simulink model "System"  (R2020a)
settings: Solver=VariableStepAuto  StartTime=0.0  StopTime=30000  RelTol=1e-3
values from neighbouring files (symbols this model uses):
  params = struct()    [LOAD_PARAMS.m]
libraries: simulink x25
(part 2 of 2)

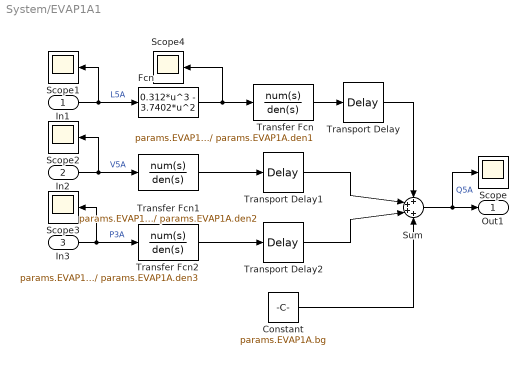
== system System/EVAP1A1 ==
  In1 : Inport
  In2 : Inport  Port=2
  In3 : Inport  Port=3
  Constant : Constant  Value=params.EVAP1A.bg
  Fcn : Fcn  Expr=0.312*u^3 - 3.7402*u^2
  Scope{,1..4} (5 alike) : Scope
  Sum : Sum  Inputs=++++
  Transfer Fcn : TransferFcn  Numerator=params.EVAP1A.num1  Denominator=params.EVAP1A.den1
  Transfer Fcn1 : TransferFcn  Numerator=params.EVAP1A.num2  Denominator=params.EVAP1A.den2
  Transfer Fcn2 : TransferFcn  Numerator=params.EVAP1A.num3  Denominator=params.EVAP1A.den3
  Transport Delay : TransportDelay  DelayTime=params.EVAP1A.td1
  Transport Delay1 : TransportDelay  DelayTime=params.EVAP1A.td2
  Transport Delay2 : TransportDelay  DelayTime=params.EVAP1A.td3
  Out1 : Outport
  wires:
  Transfer Fcn/1 -> Transport Delay/1
  Transfer Fcn1/1 -> Transport Delay1/1
  Transfer Fcn2/1 -> Transport Delay2/1
  In1/1 -> Fcn/1, Scope1/1  "L5A"
  In2/1 -> Scope2/1, Transfer Fcn1/1  "V5A"
  In3/1 -> Scope3/1, Transfer Fcn2/1  "P3A"
  Sum/1 -> Scope/1, Out1/1  "Q5A"
  Constant/1 -> Sum/4
  Fcn/1 -> Scope4/1, Transfer Fcn/1
  Transport Delay/1 -> Sum/1
  Transport Delay1/1 -> Sum/2
  Transport Delay2/1 -> Sum/3

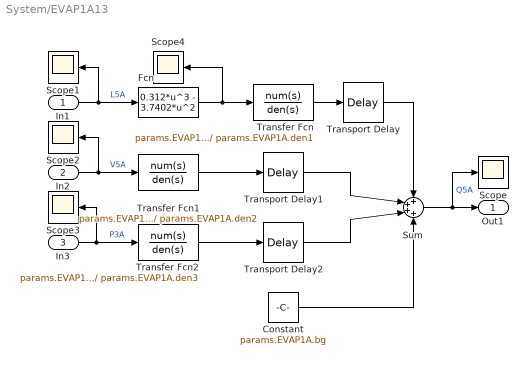
== system System/EVAP1A13 ==
  In1 : Inport
  In2 : Inport  Port=2
  In3 : Inport  Port=3
  Constant : Constant  Value=params.EVAP1A.bg
  Fcn : Fcn  Expr=0.312*u^3 - 3.7402*u^2
  Scope{,1..4} (5 alike) : Scope
  Sum : Sum  Inputs=++++
  Transfer Fcn : TransferFcn  Numerator=params.EVAP1A.num1  Denominator=params.EVAP1A.den1
  Transfer Fcn1 : TransferFcn  Numerator=params.EVAP1A.num2  Denominator=params.EVAP1A.den2
  Transfer Fcn2 : TransferFcn  Numerator=params.EVAP1A.num3  Denominator=params.EVAP1A.den3
  Transport Delay : TransportDelay  DelayTime=params.EVAP1A.td1
  Transport Delay1 : TransportDelay  DelayTime=params.EVAP1A.td2
  Transport Delay2 : TransportDelay  DelayTime=params.EVAP1A.td3
  Out1 : Outport
  wires:
  Transfer Fcn/1 -> Transport Delay/1
  Transfer Fcn1/1 -> Transport Delay1/1
  Transfer Fcn2/1 -> Transport Delay2/1
  In1/1 -> Fcn/1, Scope1/1  "L5A"
  In2/1 -> Scope2/1, Transfer Fcn1/1  "V5A"
  In3/1 -> Scope3/1, Transfer Fcn2/1  "P3A"
  Sum/1 -> Scope/1, Out1/1  "Q5A"
  Constant/1 -> Sum/4
  Fcn/1 -> Scope4/1, Transfer Fcn/1
  Transport Delay/1 -> Sum/1
  Transport Delay1/1 -> Sum/2
  Transport Delay2/1 -> Sum/3

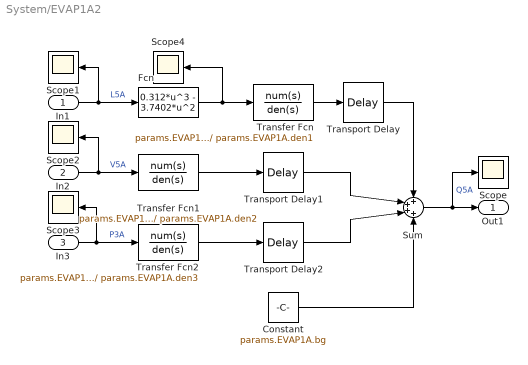
== system System/EVAP1A2 ==
  In1 : Inport
  In2 : Inport  Port=2
  In3 : Inport  Port=3
  Constant : Constant  Value=params.EVAP1A.bg
  Fcn : Fcn  Expr=0.312*u^3 - 3.7402*u^2
  Scope{,1..4} (5 alike) : Scope
  Sum : Sum  Inputs=++++
  Transfer Fcn : TransferFcn  Numerator=params.EVAP1A.num1  Denominator=params.EVAP1A.den1
  Transfer Fcn1 : TransferFcn  Numerator=params.EVAP1A.num2  Denominator=params.EVAP1A.den2
  Transfer Fcn2 : TransferFcn  Numerator=params.EVAP1A.num3  Denominator=params.EVAP1A.den3
  Transport Delay : TransportDelay  DelayTime=params.EVAP1A.td1
  Transport Delay1 : TransportDelay  DelayTime=params.EVAP1A.td2
  Transport Delay2 : TransportDelay  DelayTime=params.EVAP1A.td3
  Out1 : Outport
  wires:
  Transfer Fcn/1 -> Transport Delay/1
  Transfer Fcn1/1 -> Transport Delay1/1
  Transfer Fcn2/1 -> Transport Delay2/1
  In1/1 -> Fcn/1, Scope1/1  "L5A"
  In2/1 -> Scope2/1, Transfer Fcn1/1  "V5A"
  In3/1 -> Scope3/1, Transfer Fcn2/1  "P3A"
  Sum/1 -> Scope/1, Out1/1  "Q5A"
  Constant/1 -> Sum/4
  Fcn/1 -> Scope4/1, Transfer Fcn/1
  Transport Delay/1 -> Sum/1
  Transport Delay1/1 -> Sum/2
  Transport Delay2/1 -> Sum/3

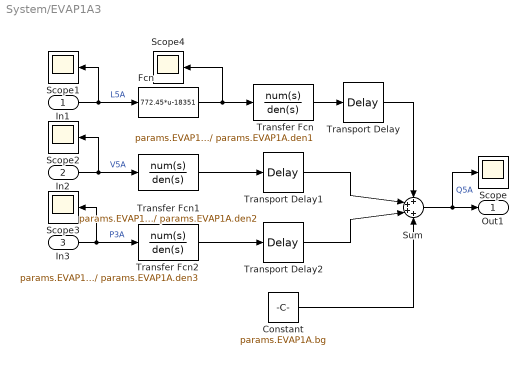
== system System/EVAP1A3 ==
  In1 : Inport
  In2 : Inport  Port=2
  In3 : Inport  Port=3
  Constant : Constant  Value=params.EVAP1A.bg
  Fcn : Fcn  Expr=772.45*u-18351
  Scope{,1..4} (5 alike) : Scope
  Sum : Sum  Inputs=++++
  Transfer Fcn : TransferFcn  Numerator=params.EVAP1A.num1  Denominator=params.EVAP1A.den1
  Transfer Fcn1 : TransferFcn  Numerator=params.EVAP1A.num2  Denominator=params.EVAP1A.den2
  Transfer Fcn2 : TransferFcn  Numerator=params.EVAP1A.num3  Denominator=params.EVAP1A.den3
  Transport Delay : TransportDelay  DelayTime=params.EVAP1A.td1
  Transport Delay1 : TransportDelay  DelayTime=params.EVAP1A.td2
  Transport Delay2 : TransportDelay  DelayTime=params.EVAP1A.td3
  Out1 : Outport
  wires:
  Transfer Fcn/1 -> Transport Delay/1
  Transfer Fcn1/1 -> Transport Delay1/1
  Transfer Fcn2/1 -> Transport Delay2/1
  In1/1 -> Fcn/1, Scope1/1  "L5A"
  In2/1 -> Scope2/1, Transfer Fcn1/1  "V5A"
  In3/1 -> Scope3/1, Transfer Fcn2/1  "P3A"
  Sum/1 -> Scope/1, Out1/1  "Q5A"
  Constant/1 -> Sum/4
  Fcn/1 -> Scope4/1, Transfer Fcn/1
  Transport Delay/1 -> Sum/1
  Transport Delay1/1 -> Sum/2
  Transport Delay2/1 -> Sum/3

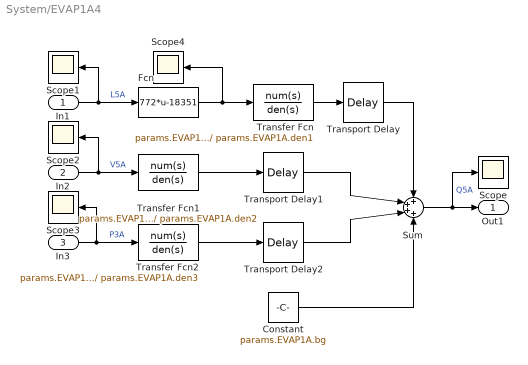
== system System/EVAP1A4 ==
  In1 : Inport
  In2 : Inport  Port=2
  In3 : Inport  Port=3
  Constant : Constant  Value=params.EVAP1A.bg
  Fcn : Fcn  Expr=772*u-18351
  Scope{,1..4} (5 alike) : Scope
  Sum : Sum  Inputs=++++
  Transfer Fcn : TransferFcn  Numerator=params.EVAP1A.num1  Denominator=params.EVAP1A.den1
  Transfer Fcn1 : TransferFcn  Numerator=params.EVAP1A.num2  Denominator=params.EVAP1A.den2
  Transfer Fcn2 : TransferFcn  Numerator=params.EVAP1A.num3  Denominator=params.EVAP1A.den3
  Transport Delay : TransportDelay  DelayTime=params.EVAP1A.td1
  Transport Delay1 : TransportDelay  DelayTime=params.EVAP1A.td2
  Transport Delay2 : TransportDelay  DelayTime=params.EVAP1A.td3
  Out1 : Outport
  wires:
  Transfer Fcn/1 -> Transport Delay/1
  Transfer Fcn1/1 -> Transport Delay1/1
  Transfer Fcn2/1 -> Transport Delay2/1
  In1/1 -> Fcn/1, Scope1/1  "L5A"
  In2/1 -> Scope2/1, Transfer Fcn1/1  "V5A"
  In3/1 -> Scope3/1, Transfer Fcn2/1  "P3A"
  Sum/1 -> Scope/1, Out1/1  "Q5A"
  Constant/1 -> Sum/4
  Fcn/1 -> Scope4/1, Transfer Fcn/1
  Transport Delay/1 -> Sum/1
  Transport Delay1/1 -> Sum/2
  Transport Delay2/1 -> Sum/3

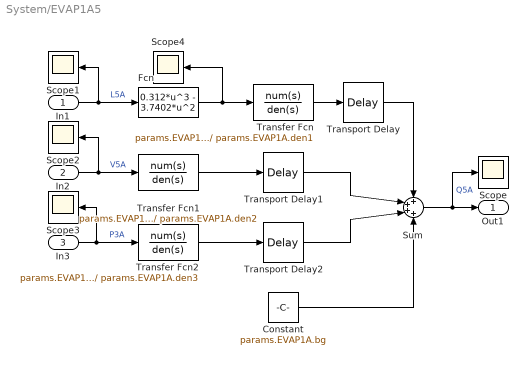
== system System/EVAP1A5 ==
  In1 : Inport
  In2 : Inport  Port=2
  In3 : Inport  Port=3
  Constant : Constant  Value=params.EVAP1A.bg
  Fcn : Fcn  Expr=0.312*u^3 - 3.7402*u^2
  Scope{,1..4} (5 alike) : Scope
  Sum : Sum  Inputs=++++
  Transfer Fcn : TransferFcn  Numerator=params.EVAP1A.num1  Denominator=params.EVAP1A.den1
  Transfer Fcn1 : TransferFcn  Numerator=params.EVAP1A.num2  Denominator=params.EVAP1A.den2
  Transfer Fcn2 : TransferFcn  Numerator=params.EVAP1A.num3  Denominator=params.EVAP1A.den3
  Transport Delay : TransportDelay  DelayTime=params.EVAP1A.td1
  Transport Delay1 : TransportDelay  DelayTime=params.EVAP1A.td2
  Transport Delay2 : TransportDelay  DelayTime=params.EVAP1A.td3
  Out1 : Outport
  wires:
  Transfer Fcn/1 -> Transport Delay/1
  Transfer Fcn1/1 -> Transport Delay1/1
  Transfer Fcn2/1 -> Transport Delay2/1
  In1/1 -> Fcn/1, Scope1/1  "L5A"
  In2/1 -> Scope2/1, Transfer Fcn1/1  "V5A"
  In3/1 -> Scope3/1, Transfer Fcn2/1  "P3A"
  Sum/1 -> Scope/1, Out1/1  "Q5A"
  Constant/1 -> Sum/4
  Fcn/1 -> Scope4/1, Transfer Fcn/1
  Transport Delay/1 -> Sum/1
  Transport Delay1/1 -> Sum/2
  Transport Delay2/1 -> Sum/3

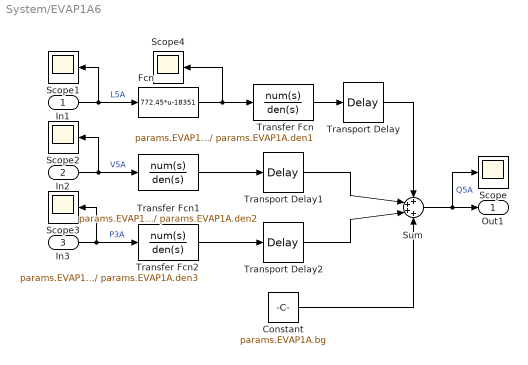
== system System/EVAP1A6 ==
  In1 : Inport
  In2 : Inport  Port=2
  In3 : Inport  Port=3
  Constant : Constant  Value=params.EVAP1A.bg
  Fcn : Fcn  Expr=772.45*u-18351
  Scope{,1..4} (5 alike) : Scope
  Sum : Sum  Inputs=++++
  Transfer Fcn : TransferFcn  Numerator=params.EVAP1A.num1  Denominator=params.EVAP1A.den1
  Transfer Fcn1 : TransferFcn  Numerator=params.EVAP1A.num2  Denominator=params.EVAP1A.den2
  Transfer Fcn2 : TransferFcn  Numerator=params.EVAP1A.num3  Denominator=params.EVAP1A.den3
  Transport Delay : TransportDelay  DelayTime=params.EVAP1A.td1
  Transport Delay1 : TransportDelay  DelayTime=params.EVAP1A.td2
  Transport Delay2 : TransportDelay  DelayTime=params.EVAP1A.td3
  Out1 : Outport
  wires:
  Transfer Fcn/1 -> Transport Delay/1
  Transfer Fcn1/1 -> Transport Delay1/1
  Transfer Fcn2/1 -> Transport Delay2/1
  In1/1 -> Fcn/1, Scope1/1  "L5A"
  In2/1 -> Scope2/1, Transfer Fcn1/1  "V5A"
  In3/1 -> Scope3/1, Transfer Fcn2/1  "P3A"
  Sum/1 -> Scope/1, Out1/1  "Q5A"
  Constant/1 -> Sum/4
  Fcn/1 -> Scope4/1, Transfer Fcn/1
  Transport Delay/1 -> Sum/1
  Transport Delay1/1 -> Sum/2
  Transport Delay2/1 -> Sum/3

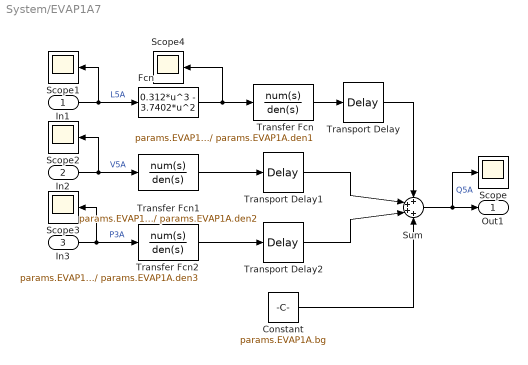
== system System/EVAP1A7 ==
  In1 : Inport
  In2 : Inport  Port=2
  In3 : Inport  Port=3
  Constant : Constant  Value=params.EVAP1A.bg
  Fcn : Fcn  Expr=0.312*u^3 - 3.7402*u^2
  Scope{,1..4} (5 alike) : Scope
  Sum : Sum  Inputs=++++
  Transfer Fcn : TransferFcn  Numerator=params.EVAP1A.num1  Denominator=params.EVAP1A.den1
  Transfer Fcn1 : TransferFcn  Numerator=params.EVAP1A.num2  Denominator=params.EVAP1A.den2
  Transfer Fcn2 : TransferFcn  Numerator=params.EVAP1A.num3  Denominator=params.EVAP1A.den3
  Transport Delay : TransportDelay  DelayTime=params.EVAP1A.td1
  Transport Delay1 : TransportDelay  DelayTime=params.EVAP1A.td2
  Transport Delay2 : TransportDelay  DelayTime=params.EVAP1A.td3
  Out1 : Outport
  wires:
  Transfer Fcn/1 -> Transport Delay/1
  Transfer Fcn1/1 -> Transport Delay1/1
  Transfer Fcn2/1 -> Transport Delay2/1
  In1/1 -> Fcn/1, Scope1/1  "L5A"
  In2/1 -> Scope2/1, Transfer Fcn1/1  "V5A"
  In3/1 -> Scope3/1, Transfer Fcn2/1  "P3A"
  Sum/1 -> Scope/1, Out1/1  "Q5A"
  Constant/1 -> Sum/4
  Fcn/1 -> Scope4/1, Transfer Fcn/1
  Transport Delay/1 -> Sum/1
  Transport Delay1/1 -> Sum/2
  Transport Delay2/1 -> Sum/3

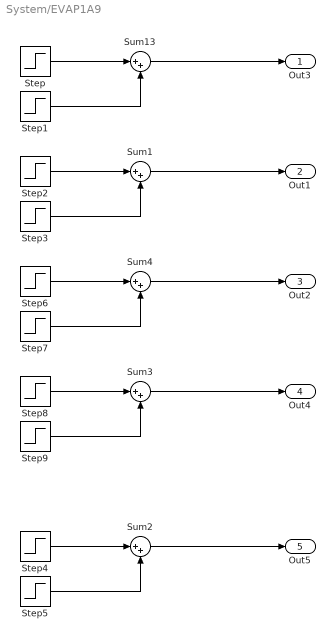
== system System/EVAP1A9 ==
  Step : Step  Time=1000  Before=200  After=0  SampleTime=0
  Step1 : Step  Time=2000  After=200  SampleTime=0
  Step2 : Step  Time=1000  Before=2  After=0  SampleTime=0
  Step3 : Step  Time=2000  After=2  SampleTime=0
  Step4 : Step  Time=1000  Before=74  After=72  SampleTime=0
  Step5 : Step  Time=2000  After=2  SampleTime=0
  Step6 : Step  Time=3000  Before=200  After=0  SampleTime=0
  Step7 : Step  Time=4000  After=200  SampleTime=0
  Step8 : Step  Time=3000  Before=2  After=0  SampleTime=0
  Step9 : Step  Time=4000  After=2  SampleTime=0
  Sum{1..4,13} (5 alike) : Sum  Inputs=|++
  Out3 : Outport
  Out1 : Outport  Port=2
  Out2 : Outport  Port=3
  Out4 : Outport  Port=4
  Out5 : Outport  Port=5
  wires:
  Step1/1 -> Sum13/2
  Step/1 -> Sum13/1
  Sum13/1 -> Out3/1
  Step2/1 -> Sum1/1
  Sum1/1 -> Out1/1
  Step3/1 -> Sum1/2
  Step4/1 -> Sum2/1
  Sum2/1 -> Out5/1
  Step5/1 -> Sum2/2
  Sum4/1 -> Out2/1
  Step6/1 -> Sum4/1
  Step9/1 -> Sum3/2
  Step8/1 -> Sum3/1
  Sum3/1 -> Out4/1
  Step7/1 -> Sum4/2

== system System/EVAP2A ==
  In1 : Inport
  In2 : Inport  Port=2
  In3 : Inport  Port=3
  Constant : Constant  Value=params.EVAP1A.bg
  Fcn : Fcn  Expr=0.312*u^3 - 3.7402*u^2
  Scope{,1..3} (4 alike) : Scope
  Sum : Sum  Inputs=++++
  Transfer Fcn : TransferFcn  Numerator=params.EVAP1A.num1  Denominator=params.EVAP1A.den1
  Transfer Fcn1 : TransferFcn  Numerator=params.EVAP1A.num2  Denominator=params.EVAP1A.den2
  Transfer Fcn2 : TransferFcn  Numerator=params.EVAP1A.num3  Denominator=params.EVAP1A.den3
  Transport Delay : TransportDelay  DelayTime=params.EVAP1A.td1
  Transport Delay1 : TransportDelay  DelayTime=params.EVAP1A.td3
  Transport Delay2 : TransportDelay  DelayTime=params.EVAP1A.td2
  Out1 : Outport
  wires:
  Transfer Fcn/1 -> Transport Delay/1
  Transfer Fcn1/1 -> Transport Delay2/1
  Transfer Fcn2/1 -> Transport Delay1/1
  In1/1 -> Fcn/1, Scope1/1  "L6A"
  In2/1 -> Scope2/1, Transfer Fcn1/1  "V6A"
  In3/1 -> Scope3/1, Transfer Fcn2/1  "P3A"
  Sum/1 -> Scope/1, Out1/1  "Q5A"
  Constant/1 -> Sum/4
  Fcn/1 -> Transfer Fcn/1
  Transport Delay/1 -> Sum/1
  Transport Delay2/1 -> Sum/2
  Transport Delay1/1 -> Sum/3

== system System/EVAP2A1 ==
  In1 : Inport
  In2 : Inport  Port=2
  In3 : Inport  Port=3
  Constant : Constant  Value=params.EVAP1A.bg
  Fcn : Fcn  Expr=0.312*u^3 - 3.7402*u^2
  Scope{,1..3} (4 alike) : Scope
  Sum : Sum  Inputs=++++
  Transfer Fcn : TransferFcn  Numerator=params.EVAP1A.num1  Denominator=params.EVAP1A.den1
  Transfer Fcn1 : TransferFcn  Numerator=params.EVAP1A.num2  Denominator=params.EVAP1A.den2
  Transfer Fcn2 : TransferFcn  Numerator=params.EVAP1A.num3  Denominator=params.EVAP1A.den3
  Transport Delay : TransportDelay  DelayTime=params.EVAP1A.td1
  Transport Delay1 : TransportDelay  DelayTime=params.EVAP1A.td3
  Transport Delay2 : TransportDelay  DelayTime=params.EVAP1A.td2
  Out1 : Outport
  wires:
  Transfer Fcn/1 -> Transport Delay/1
  Transfer Fcn1/1 -> Transport Delay2/1
  Transfer Fcn2/1 -> Transport Delay1/1
  In1/1 -> Fcn/1, Scope1/1  "L6A"
  In2/1 -> Scope2/1, Transfer Fcn1/1  "V6A"
  In3/1 -> Scope3/1, Transfer Fcn2/1  "P3A"
  Sum/1 -> Scope/1, Out1/1  "Q5A"
  Constant/1 -> Sum/4
  Fcn/1 -> Transfer Fcn/1
  Transport Delay/1 -> Sum/1
  Transport Delay2/1 -> Sum/2
  Transport Delay1/1 -> Sum/3

== system System/EVAP2A3 ==
  In1 : Inport
  In2 : Inport  Port=2
  In3 : Inport  Port=3
  Constant : Constant  Value=params.EVAP1A.bg
  Fcn : Fcn  Expr=772.45*u-18351
  Scope{,1..3} (4 alike) : Scope
  Sum : Sum  Inputs=++++
  Transfer Fcn : TransferFcn  Numerator=params.EVAP1A.num1  Denominator=params.EVAP1A.den1
  Transfer Fcn1 : TransferFcn  Numerator=params.EVAP1A.num2  Denominator=params.EVAP1A.den2
  Transfer Fcn2 : TransferFcn  Numerator=params.EVAP1A.num3  Denominator=params.EVAP1A.den3
  Transport Delay : TransportDelay  DelayTime=params.EVAP1A.td1
  Transport Delay1 : TransportDelay  DelayTime=params.EVAP1A.td3
  Transport Delay2 : TransportDelay  DelayTime=params.EVAP1A.td2
  Out1 : Outport
  wires:
  Transfer Fcn/1 -> Transport Delay/1
  Transfer Fcn1/1 -> Transport Delay2/1
  Transfer Fcn2/1 -> Transport Delay1/1
  In1/1 -> Fcn/1, Scope1/1  "L6A"
  In2/1 -> Scope2/1, Transfer Fcn1/1  "V6A"
  In3/1 -> Scope3/1, Transfer Fcn2/1  "P3A"
  Sum/1 -> Scope/1, Out1/1  "Q5A"
  Constant/1 -> Sum/4
  Fcn/1 -> Transfer Fcn/1
  Transport Delay/1 -> Sum/1
  Transport Delay2/1 -> Sum/2
  Transport Delay1/1 -> Sum/3

== system System/EVAP2A4 ==
  In1 : Inport
  In2 : Inport  Port=2
  In3 : Inport  Port=3
  Constant : Constant  Value=params.EVAP1A.bg
  Fcn : Fcn  Expr=772.45*u-18351
  Scope{,1..3} (4 alike) : Scope
  Sum : Sum  Inputs=++++
  Transfer Fcn : TransferFcn  Numerator=params.EVAP1A.num1  Denominator=params.EVAP1A.den1
  Transfer Fcn1 : TransferFcn  Numerator=params.EVAP1A.num2  Denominator=params.EVAP1A.den2
  Transfer Fcn2 : TransferFcn  Numerator=params.EVAP1A.num3  Denominator=params.EVAP1A.den3
  Transport Delay : TransportDelay  DelayTime=params.EVAP1A.td1
  Transport Delay1 : TransportDelay  DelayTime=params.EVAP1A.td3
  Transport Delay2 : TransportDelay  DelayTime=params.EVAP1A.td2
  Out1 : Outport
  wires:
  Transfer Fcn/1 -> Transport Delay/1
  Transfer Fcn1/1 -> Transport Delay2/1
  Transfer Fcn2/1 -> Transport Delay1/1
  In1/1 -> Fcn/1, Scope1/1  "L6A"
  In2/1 -> Scope2/1, Transfer Fcn1/1  "V6A"
  In3/1 -> Scope3/1, Transfer Fcn2/1  "P3A"
  Sum/1 -> Scope/1, Out1/1  "Q5A"
  Constant/1 -> Sum/4
  Fcn/1 -> Transfer Fcn/1
  Transport Delay/1 -> Sum/1
  Transport Delay2/1 -> Sum/2
  Transport Delay1/1 -> Sum/3

== system System/EVAP2A5 ==
  In1 : Inport
  In2 : Inport  Port=2
  In3 : Inport  Port=3
  Constant : Constant  Value=params.EVAP1A.bg
  Fcn : Fcn  Expr=0.312*u^3 - 3.7402*u^2
  Scope{,1..3} (4 alike) : Scope
  Sum : Sum  Inputs=++++
  Transfer Fcn : TransferFcn  Numerator=params.EVAP1A.num1  Denominator=params.EVAP1A.den1
  Transfer Fcn1 : TransferFcn  Numerator=params.EVAP1A.num2  Denominator=params.EVAP1A.den2
  Transfer Fcn2 : TransferFcn  Numerator=params.EVAP1A.num3  Denominator=params.EVAP1A.den3
  Transport Delay : TransportDelay  DelayTime=params.EVAP1A.td1
  Transport Delay1 : TransportDelay  DelayTime=params.EVAP1A.td3
  Transport Delay2 : TransportDelay  DelayTime=params.EVAP1A.td2
  Out1 : Outport
  wires:
  Transfer Fcn/1 -> Transport Delay/1
  Transfer Fcn1/1 -> Transport Delay2/1
  Transfer Fcn2/1 -> Transport Delay1/1
  In1/1 -> Fcn/1, Scope1/1  "L6A"
  In2/1 -> Scope2/1, Transfer Fcn1/1  "V6A"
  In3/1 -> Scope3/1, Transfer Fcn2/1  "P3A"
  Sum/1 -> Scope/1, Out1/1  "Q5A"
  Constant/1 -> Sum/4
  Fcn/1 -> Transfer Fcn/1
  Transport Delay/1 -> Sum/1
  Transport Delay2/1 -> Sum/2
  Transport Delay1/1 -> Sum/3

== system System/EVAP2A6 ==
  In1 : Inport
  In2 : Inport  Port=2
  In3 : Inport  Port=3
  Constant : Constant  Value=params.EVAP1A.bg
  Fcn : Fcn  Expr=772.45*u-18351
  Scope{,1..3} (4 alike) : Scope
  Sum : Sum  Inputs=++++
  Transfer Fcn : TransferFcn  Numerator=params.EVAP1A.num1  Denominator=params.EVAP1A.den1
  Transfer Fcn1 : TransferFcn  Numerator=params.EVAP1A.num2  Denominator=params.EVAP1A.den2
  Transfer Fcn2 : TransferFcn  Numerator=params.EVAP1A.num3  Denominator=params.EVAP1A.den3
  Transport Delay : TransportDelay  DelayTime=params.EVAP1A.td1
  Transport Delay1 : TransportDelay  DelayTime=params.EVAP1A.td3
  Transport Delay2 : TransportDelay  DelayTime=params.EVAP1A.td2
  Out1 : Outport
  wires:
  Transfer Fcn/1 -> Transport Delay/1
  Transfer Fcn1/1 -> Transport Delay2/1
  Transfer Fcn2/1 -> Transport Delay1/1
  In1/1 -> Fcn/1, Scope1/1  "L6A"
  In2/1 -> Scope2/1, Transfer Fcn1/1  "V6A"
  In3/1 -> Scope3/1, Transfer Fcn2/1  "P3A"
  Sum/1 -> Scope/1, Out1/1  "Q5A"
  Constant/1 -> Sum/4
  Fcn/1 -> Transfer Fcn/1
  Transport Delay/1 -> Sum/1
  Transport Delay2/1 -> Sum/2
  Transport Delay1/1 -> Sum/3

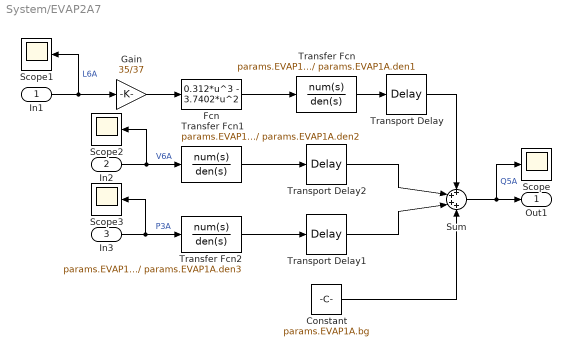
== system System/EVAP2A7 ==
  In1 : Inport
  In2 : Inport  Port=2
  In3 : Inport  Port=3
  Constant : Constant  Value=params.EVAP1A.bg
  Fcn : Fcn  Expr=0.312*u^3 - 3.7402*u^2
  Gain : Gain  Gain=35/37
  Scope{,1..3} (4 alike) : Scope
  Sum : Sum  Inputs=++++
  Transfer Fcn : TransferFcn  Numerator=params.EVAP1A.num1  Denominator=params.EVAP1A.den1
  Transfer Fcn1 : TransferFcn  Numerator=params.EVAP1A.num2  Denominator=params.EVAP1A.den2
  Transfer Fcn2 : TransferFcn  Numerator=params.EVAP1A.num3  Denominator=params.EVAP1A.den3
  Transport Delay : TransportDelay  DelayTime=params.EVAP1A.td1
  Transport Delay1 : TransportDelay  DelayTime=params.EVAP1A.td3
  Transport Delay2 : TransportDelay  DelayTime=params.EVAP1A.td2
  Out1 : Outport
  wires:
  Transfer Fcn/1 -> Transport Delay/1
  Transfer Fcn1/1 -> Transport Delay2/1
  Transfer Fcn2/1 -> Transport Delay1/1
  In1/1 -> Gain/1, Scope1/1  "L6A"
  In2/1 -> Scope2/1, Transfer Fcn1/1  "V6A"
  In3/1 -> Scope3/1, Transfer Fcn2/1  "P3A"
  Sum/1 -> Scope/1, Out1/1  "Q5A"
  Constant/1 -> Sum/4
  Fcn/1 -> Transfer Fcn/1
  Transport Delay/1 -> Sum/1
  Transport Delay2/1 -> Sum/2
  Transport Delay1/1 -> Sum/3
  Gain/1 -> Fcn/1

== system System/FILTERA ==
  In1 : Inport
  In2 : Inport  Port=2
  Constant : Constant  Value=params.FILTERA.bg
  Scope : Scope
  Scope1 : Scope
  Scope2 : Scope
  Sum : Sum  Inputs=+++
  Transfer Fcn : TransferFcn  Numerator=params.FILTERA.num1  Denominator=params.FILTERA.den1
  Transfer Fcn1 : TransferFcn  Numerator=params.FILTERA.num2  Denominator=params.FILTERA.den2
  Transport Delay : TransportDelay  DelayTime=params.FILTERA.td1
  Transport Delay1 : TransportDelay  DelayTime=params.FILTERA.td2
  Out1 : Outport
  wires:
  Transfer Fcn/1 -> Transport Delay/1
  Transfer Fcn1/1 -> Transport Delay1/1
  In1/1 -> Scope1/1, Transfer Fcn/1  "P2A"
  In2/1 -> Scope2/1, Transfer Fcn1/1  "Q"
  Sum/1 -> Scope/1, Out1/1  "P3A"
  Constant/1 -> Sum/3
  Transport Delay/1 -> Sum/1
  Transport Delay1/1 -> Sum/2

== system System/FILTERA1 ==
  In1 : Inport
  In2 : Inport  Port=2
  Constant : Constant  Value=params.FILTERA.bg
  Scope : Scope
  Scope1 : Scope
  Scope2 : Scope
  Sum : Sum  Inputs=+++
  Transfer Fcn : TransferFcn  Numerator=params.FILTERA.num1  Denominator=params.FILTERA.den1
  Transfer Fcn1 : TransferFcn  Numerator=params.FILTERA.num2  Denominator=params.FILTERA.den2
  Transport Delay : TransportDelay  DelayTime=params.FILTERA.td1
  Transport Delay1 : TransportDelay  DelayTime=params.FILTERA.td2
  Out1 : Outport
  wires:
  Transfer Fcn/1 -> Transport Delay/1
  Transfer Fcn1/1 -> Transport Delay1/1
  In1/1 -> Scope1/1, Transfer Fcn/1  "P2A"
  In2/1 -> Scope2/1, Transfer Fcn1/1  "Q"
  Sum/1 -> Scope/1, Out1/1  "P3A"
  Constant/1 -> Sum/3
  Transport Delay/1 -> Sum/1
  Transport Delay1/1 -> Sum/2

== system System/FILTERA2 ==
  In1 : Inport
  In2 : Inport  Port=2
  Constant : Constant  Value=params.FILTERA.bg
  Scope : Scope
  Scope1 : Scope
  Scope2 : Scope
  Sum : Sum  Inputs=+++
  Transfer Fcn : TransferFcn  Numerator=params.FILTERA.num1  Denominator=params.FILTERA.den1
  Transfer Fcn1 : TransferFcn  Numerator=params.FILTERA.num2  Denominator=params.FILTERA.den2
  Transport Delay : TransportDelay  DelayTime=params.FILTERA.td1
  Transport Delay1 : TransportDelay  DelayTime=params.FILTERA.td2
  Out1 : Outport
  wires:
  Transfer Fcn/1 -> Transport Delay/1
  Transfer Fcn1/1 -> Transport Delay1/1
  In1/1 -> Scope1/1, Transfer Fcn/1  "P2A"
  In2/1 -> Scope2/1, Transfer Fcn1/1  "Q"
  Sum/1 -> Scope/1, Out1/1  "P3A"
  Constant/1 -> Sum/3
  Transport Delay/1 -> Sum/1
  Transport Delay1/1 -> Sum/2

== system System/FILTERA3 ==
  In1 : Inport
  In2 : Inport  Port=2
  Constant : Constant  Value=params.FILTERA.bg
  Scope : Scope
  Scope1 : Scope
  Scope2 : Scope
  Sum : Sum  Inputs=+++
  Transfer Fcn : TransferFcn  Numerator=params.FILTERA.num1  Denominator=params.FILTERA.den1
  Transfer Fcn1 : TransferFcn  Numerator=params.FILTERA.num2  Denominator=params.FILTERA.den2
  Transport Delay : TransportDelay  DelayTime=params.FILTERA.td1
  Transport Delay1 : TransportDelay  DelayTime=params.FILTERA.td2
  Out1 : Outport
  wires:
  Transfer Fcn/1 -> Transport Delay/1
  Transfer Fcn1/1 -> Transport Delay1/1
  In1/1 -> Scope1/1, Transfer Fcn/1  "P2A"
  In2/1 -> Scope2/1, Transfer Fcn1/1  "Q"
  Sum/1 -> Scope/1, Out1/1  "P3A"
  Constant/1 -> Sum/3
  Transport Delay/1 -> Sum/1
  Transport Delay1/1 -> Sum/2

== system System/FILTERA4 ==
  In1 : Inport
  In2 : Inport  Port=2
  Constant : Constant  Value=params.FILTERA.bg
  Scope : Scope
  Scope1 : Scope
  Scope2 : Scope
  Sum : Sum  Inputs=+++
  Transfer Fcn : TransferFcn  Numerator=params.FILTERA.num1  Denominator=params.FILTERA.den1
  Transfer Fcn1 : TransferFcn  Numerator=params.FILTERA.num2  Denominator=params.FILTERA.den2
  Transport Delay : TransportDelay  DelayTime=params.FILTERA.td1
  Transport Delay1 : TransportDelay  DelayTime=params.FILTERA.td2
  Out1 : Outport
  wires:
  Transfer Fcn/1 -> Transport Delay/1
  Transfer Fcn1/1 -> Transport Delay1/1
  In1/1 -> Scope1/1, Transfer Fcn/1  "P2A"
  In2/1 -> Scope2/1, Transfer Fcn1/1  "Q"
  Sum/1 -> Scope/1, Out1/1  "P3A"
  Constant/1 -> Sum/3
  Transport Delay/1 -> Sum/1
  Transport Delay1/1 -> Sum/2

== system System/FILTERA5 ==
  In1 : Inport
  In2 : Inport  Port=2
  Constant : Constant  Value=params.FILTERA.bg
  Scope : Scope
  Scope1 : Scope
  Scope2 : Scope
  Sum : Sum  Inputs=+++
  Transfer Fcn : TransferFcn  Numerator=params.FILTERA.num1  Denominator=params.FILTERA.den1
  Transfer Fcn1 : TransferFcn  Numerator=params.FILTERA.num2  Denominator=params.FILTERA.den2
  Transport Delay : TransportDelay  DelayTime=params.FILTERA.td1
  Transport Delay1 : TransportDelay  DelayTime=params.FILTERA.td2
  Out1 : Outport
  wires:
  Transfer Fcn/1 -> Transport Delay/1
  Transfer Fcn1/1 -> Transport Delay1/1
  In1/1 -> Scope1/1, Transfer Fcn/1  "P2A"
  In2/1 -> Scope2/1, Transfer Fcn1/1  "Q"
  Sum/1 -> Scope/1, Out1/1  "P3A"
  Constant/1 -> Sum/3
  Transport Delay/1 -> Sum/1
  Transport Delay1/1 -> Sum/2

== system System/FILTERA6 ==
  In1 : Inport
  In2 : Inport  Port=2
  Constant : Constant  Value=params.FILTERA.bg
  Scope : Scope
  Scope1 : Scope
  Scope2 : Scope
  Sum : Sum  Inputs=+++
  Transfer Fcn : TransferFcn  Numerator=params.FILTERA.num1  Denominator=params.FILTERA.den1
  Transfer Fcn1 : TransferFcn  Numerator=params.FILTERA.num2  Denominator=params.FILTERA.den2
  Transport Delay : TransportDelay  DelayTime=params.FILTERA.td1
  Transport Delay1 : TransportDelay  DelayTime=params.FILTERA.td2
  Out1 : Outport
  wires:
  Transfer Fcn/1 -> Transport Delay/1
  Transfer Fcn1/1 -> Transport Delay1/1
  In1/1 -> Scope1/1, Transfer Fcn/1  "P2A"
  In2/1 -> Scope2/1, Transfer Fcn1/1  "Q"
  Sum/1 -> Scope/1, Out1/1  "P3A"
  Constant/1 -> Sum/3
  Transport Delay/1 -> Sum/1
  Transport Delay1/1 -> Sum/2

== system System/FILTERA8 ==
  In1 : Inport
  In2 : Inport  Port=2
  Constant : Constant  Value=params.FILTERA.bg
  Scope : Scope
  Scope1 : Scope
  Scope2 : Scope
  Sum : Sum  Inputs=+++
  Transfer Fcn : TransferFcn  Numerator=params.FILTERA.num1  Denominator=params.FILTERA.den1
  Transfer Fcn1 : TransferFcn  Numerator=params.FILTERA.num2  Denominator=params.FILTERA.den2
  Transport Delay : TransportDelay  DelayTime=params.FILTERA.td1
  Transport Delay1 : TransportDelay  DelayTime=params.FILTERA.td2
  Out1 : Outport
  wires:
  Transfer Fcn/1 -> Transport Delay/1
  Transfer Fcn1/1 -> Transport Delay1/1
  In1/1 -> Scope1/1, Transfer Fcn/1  "P2A"
  In2/1 -> Scope2/1, Transfer Fcn1/1  "Q"
  Sum/1 -> Scope/1, Out1/1  "P3A"
  Constant/1 -> Sum/3
  Transport Delay/1 -> Sum/1
  Transport Delay1/1 -> Sum/2

== system System/HTFA ==
  In2 : Inport
  Constant : Constant  Value=params.HTFA.bg
  Scope : Scope
  Scope1 : Scope
  Sum : Sum  Inputs=|++
  Transfer Fcn1 : TransferFcn  Numerator=params.HTFA.num1  Denominator=params.HTFA.den1
  Transport Delay : TransportDelay  DelayTime=params.HTFA.td1
  Out1 : Outport
  wires:
  In2/1 -> Scope1/1, Transfer Fcn1/1  "P3A"
  Transfer Fcn1/1 -> Transport Delay/1
  Sum/1 -> Scope/1, Out1/1  "Q4A"
  Constant/1 -> Sum/2
  Transport Delay/1 -> Sum/1

== system System/HTFA1 ==
  In2 : Inport
  Constant : Constant  Value=params.HTFA.bg
  Scope : Scope
  Scope1 : Scope
  Sum : Sum  Inputs=|++
  Transfer Fcn1 : TransferFcn  Numerator=params.HTFA.num1  Denominator=params.HTFA.den1
  Transport Delay : TransportDelay  DelayTime=params.HTFA.td1
  Out1 : Outport
  wires:
  In2/1 -> Scope1/1, Transfer Fcn1/1  "P3A"
  Transfer Fcn1/1 -> Transport Delay/1
  Sum/1 -> Scope/1, Out1/1  "Q4A"
  Constant/1 -> Sum/2
  Transport Delay/1 -> Sum/1

== system System/HTFA2 ==
  In2 : Inport
  Constant : Constant  Value=params.HTFA.bg
  Scope : Scope
  Scope1 : Scope
  Sum : Sum  Inputs=|++
  Transfer Fcn1 : TransferFcn  Numerator=params.HTFA.num1  Denominator=params.HTFA.den1
  Transport Delay : TransportDelay  DelayTime=params.HTFA.td1
  Out1 : Outport
  wires:
  In2/1 -> Scope1/1, Transfer Fcn1/1  "P3A"
  Transfer Fcn1/1 -> Transport Delay/1
  Sum/1 -> Scope/1, Out1/1  "Q4A"
  Constant/1 -> Sum/2
  Transport Delay/1 -> Sum/1

== system System/HTFA3 ==
  In2 : Inport
  Constant : Constant  Value=params.HTFA.bg
  Scope : Scope
  Scope1 : Scope
  Sum : Sum  Inputs=|++
  Transfer Fcn1 : TransferFcn  Numerator=params.HTFA.num1  Denominator=params.HTFA.den1
  Transport Delay : TransportDelay  DelayTime=params.HTFA.td1
  Out1 : Outport
  wires:
  In2/1 -> Scope1/1, Transfer Fcn1/1  "P3A"
  Transfer Fcn1/1 -> Transport Delay/1
  Sum/1 -> Scope/1, Out1/1  "Q4A"
  Constant/1 -> Sum/2
  Transport Delay/1 -> Sum/1

== system System/HTFA4 ==
  In2 : Inport
  Constant : Constant  Value=params.HTFA.bg
  Scope : Scope
  Scope1 : Scope
  Sum : Sum  Inputs=|++
  Transfer Fcn1 : TransferFcn  Numerator=params.HTFA.num1  Denominator=params.HTFA.den1
  Transport Delay : TransportDelay  DelayTime=params.HTFA.td1
  Out1 : Outport
  wires:
  In2/1 -> Scope1/1, Transfer Fcn1/1  "P3A"
  Transfer Fcn1/1 -> Transport Delay/1
  Sum/1 -> Scope/1, Out1/1  "Q4A"
  Constant/1 -> Sum/2
  Transport Delay/1 -> Sum/1

== system System/HTFA5 ==
  In2 : Inport
  Constant : Constant  Value=params.HTFA.bg
  Scope : Scope
  Scope1 : Scope
  Sum : Sum  Inputs=|++
  Transfer Fcn1 : TransferFcn  Numerator=params.HTFA.num1  Denominator=params.HTFA.den1
  Transport Delay : TransportDelay  DelayTime=params.HTFA.td1
  Out1 : Outport
  wires:
  In2/1 -> Scope1/1, Transfer Fcn1/1  "P3A"
  Transfer Fcn1/1 -> Transport Delay/1
  Sum/1 -> Scope/1, Out1/1  "Q4A"
  Constant/1 -> Sum/2
  Transport Delay/1 -> Sum/1

== system System/HTFA6 ==
  In2 : Inport
  Constant : Constant  Value=params.HTFA.bg
  Scope : Scope
  Scope1 : Scope
  Sum : Sum  Inputs=|++
  Transfer Fcn1 : TransferFcn  Numerator=params.HTFA.num1  Denominator=params.HTFA.den1
  Transport Delay : TransportDelay  DelayTime=params.HTFA.td1
  Out1 : Outport
  wires:
  In2/1 -> Scope1/1, Transfer Fcn1/1  "P3A"
  Transfer Fcn1/1 -> Transport Delay/1
  Sum/1 -> Scope/1, Out1/1  "Q4A"
  Constant/1 -> Sum/2
  Transport Delay/1 -> Sum/1

== system System/HTFA8 ==
  In2 : Inport
  Constant : Constant  Value=params.HTFA.bg-120
  Scope : Scope
  Scope1 : Scope
  Sum : Sum  Inputs=|++
  Transfer Fcn1 : TransferFcn  Numerator=params.HTFA.num1  Denominator=params.HTFA.den1
  Transport Delay : TransportDelay  DelayTime=params.HTFA.td1
  Out1 : Outport
  wires:
  In2/1 -> Scope1/1, Transfer Fcn1/1  "P3A"
  Transfer Fcn1/1 -> Transport Delay/1
  Sum/1 -> Scope/1, Out1/1  "Q4A"
  Constant/1 -> Sum/2
  Transport Delay/1 -> Sum/1

== system System/HTL ==
  In2 : Inport
  Constant : Constant  Value=params.HTL.bg
  Gain : Gain  Gain=2
  Scope : Scope
  Scope1 : Scope
  Sum : Sum  Inputs=|++
  Transfer Fcn1 : TransferFcn  Numerator=params.HTL.num1  Denominator=params.HTL.den1
  Transport Delay : TransportDelay  DelayTime=params.HTL.td1
  Out1 : Outport
  wires:
  In2/1 -> Scope1/1, Gain/1  "Q4A"
  Transfer Fcn1/1 -> Transport Delay/1
  Sum/1 -> Scope/1, Out1/1  "Y"
  Constant/1 -> Sum/2
  Transport Delay/1 -> Sum/1
  Gain/1 -> Transfer Fcn1/1

== system System/HTL1 ==
  In2 : Inport
  Constant : Constant  Value=params.HTL.bg
  Gain : Gain  Gain=2
  Scope : Scope
  Scope1 : Scope
  Sum : Sum  Inputs=|++
  Transfer Fcn1 : TransferFcn  Numerator=params.HTL.num1  Denominator=params.HTL.den1
  Transport Delay : TransportDelay  DelayTime=params.HTL.td1
  Out1 : Outport
  wires:
  In2/1 -> Scope1/1, Gain/1  "Q4A"
  Transfer Fcn1/1 -> Transport Delay/1
  Sum/1 -> Scope/1, Out1/1  "Y"
  Constant/1 -> Sum/2
  Transport Delay/1 -> Sum/1
  Gain/1 -> Transfer Fcn1/1

== system System/HTL2 ==
  In2 : Inport
  Constant : Constant  Value=params.HTL.bg
  Gain : Gain  Gain=2
  Scope : Scope
  Scope1 : Scope
  Sum : Sum  Inputs=|++
  Transfer Fcn1 : TransferFcn  Numerator=params.HTL.num1  Denominator=params.HTL.den1
  Transport Delay : TransportDelay  DelayTime=params.HTL.td1
  Out1 : Outport
  wires:
  In2/1 -> Scope1/1, Gain/1  "Q4A"
  Transfer Fcn1/1 -> Transport Delay/1
  Sum/1 -> Scope/1, Out1/1  "Y"
  Constant/1 -> Sum/2
  Transport Delay/1 -> Sum/1
  Gain/1 -> Transfer Fcn1/1

== system System/HTL3 ==
  In2 : Inport
  Constant : Constant  Value=params.HTL.bg
  Scope : Scope
  Scope1 : Scope
  Sum : Sum  Inputs=|++
  Transfer Fcn1 : TransferFcn  Numerator=params.HTL.num1  Denominator=params.HTL.den1
  Transport Delay : TransportDelay  DelayTime=params.HTL.td1
  Out1 : Outport
  wires:
  In2/1 -> Scope1/1, Transfer Fcn1/1  "Q4A"
  Transfer Fcn1/1 -> Transport Delay/1
  Sum/1 -> Scope/1, Out1/1  "Y"
  Constant/1 -> Sum/2
  Transport Delay/1 -> Sum/1

== system System/HTL4 ==
  In2 : Inport
  Constant : Constant  Value=params.HTL.bg
  Scope : Scope
  Scope1 : Scope
  Sum : Sum  Inputs=|++
  Transfer Fcn1 : TransferFcn  Numerator=params.HTL.num1  Denominator=params.HTL.den1
  Transport Delay : TransportDelay  DelayTime=params.HTL.td1
  Out1 : Outport
  wires:
  In2/1 -> Scope1/1, Transfer Fcn1/1  "Q4A"
  Transfer Fcn1/1 -> Transport Delay/1
  Sum/1 -> Scope/1, Out1/1  "Y"
  Constant/1 -> Sum/2
  Transport Delay/1 -> Sum/1

== system System/HTL5 ==
  In2 : Inport
  In1 : Inport  Port=2
  Constant : Constant  Value=params.HTL.bg
  Scope : Scope
  Scope1 : Scope
  Scope2 : Scope
  Sum : Sum  Inputs=|++
  Sum1 : Sum  Inputs=|++
  Transfer Fcn1 : TransferFcn  Numerator=params.HTL.num1  Denominator=params.HTL.den1
  Transport Delay : TransportDelay  DelayTime=params.HTL.td1
  Out1 : Outport
  wires:
  In2/1 -> Sum1/1, Scope1/1  "Q4A"
  Transfer Fcn1/1 -> Transport Delay/1
  Sum/1 -> Scope/1, Out1/1  "Y"
  Constant/1 -> Sum/2
  Transport Delay/1 -> Sum/1
  In1/1 -> Scope2/1, Sum1/2
  Sum1/1 -> Transfer Fcn1/1  "Y"

== system System/HTL6 ==
  In2 : Inport
  Constant : Constant  Value=params.HTL.bg
  Scope : Scope
  Scope1 : Scope
  Sum : Sum  Inputs=|++
  Transfer Fcn1 : TransferFcn  Numerator=params.HTL.num1  Denominator=params.HTL.den1
  Transport Delay : TransportDelay  DelayTime=params.HTL.td1
  Out1 : Outport
  wires:
  In2/1 -> Scope1/1, Transfer Fcn1/1  "Q4A"
  Transfer Fcn1/1 -> Transport Delay/1
  Sum/1 -> Scope/1, Out1/1  "Y"
  Constant/1 -> Sum/2
  Transport Delay/1 -> Sum/1

== system System/HTL8 ==
  In2 : Inport
  In1 : Inport  Port=2
  Constant : Constant  Value=params.HTL.bg
  Scope : Scope
  Scope1 : Scope
  Sum : Sum  Inputs=|++
  Sum1 : Sum  Inputs=|++
  Transfer Fcn1 : TransferFcn  Numerator=params.HTL.num1  Denominator=params.HTL.den1
  Transport Delay : TransportDelay  DelayTime=params.HTL.td1
  Out1 : Outport
  wires:
  In2/1 -> Sum1/1, Scope1/1  "Q4A"
  Transfer Fcn1/1 -> Transport Delay/1
  Sum/1 -> Scope/1, Out1/1  "Y"
  Constant/1 -> Sum/2
  Transport Delay/1 -> Sum/1
  In1/1 -> Sum1/2
  Sum1/1 -> Transfer Fcn1/1  "Y"

== system System/POMPAA ==
  In1 : Inport
  In2 : Inport  Port=2
  In3 : Inport  Port=3
  Constant : Constant  Value=params.POMPAA.bg
  Scope{1..4} (4 alike) : Scope
  Sum : Sum  Inputs=++++
  Transfer Fcn : TransferFcn  Numerator=params.POMPAA.num1  Denominator=params.POMPAA.den1
  Transfer Fcn1 : TransferFcn  Numerator=params.POMPAA.num2  Denominator=params.POMPAA.den2
  Transfer Fcn2 : TransferFcn  Numerator=params.POMPAA.num3  Denominator=params.POMPAA.den3
  Transport Delay : TransportDelay  DelayTime=params.POMPAA.td1
  Transport Delay1 : TransportDelay  DelayTime=params.POMPAA.td2
  Transport Delay2 : TransportDelay  DelayTime=params.POMPAA.td3
  Out1 : Outport
  wires:
  Transfer Fcn/1 -> Transport Delay/1
  Transfer Fcn1/1 -> Transport Delay1/1
  Transfer Fcn2/1 -> Transport Delay2/1
  In1/1 -> Scope2/1, Transfer Fcn/1  "omega_casA"
  In2/1 -> Scope1/1, Transfer Fcn1/1  "omega_manA"
  In3/1 -> Scope4/1, Transfer Fcn2/1  "Q"
  Sum/1 -> Scope3/1, Out1/1  "Q5A"
  Constant/1 -> Sum/4
  Transport Delay/1 -> Sum/1
  Transport Delay1/1 -> Sum/2
  Transport Delay2/1 -> Sum/3

== system System/POMPAA1 ==
  In1 : Inport
  In2 : Inport  Port=2
  In3 : Inport  Port=3
  Constant : Constant  Value=params.POMPAA.bg
  Scope{1..4} (4 alike) : Scope
  Sum : Sum  Inputs=++++
  Transfer Fcn : TransferFcn  Numerator=params.POMPAA.num1  Denominator=params.POMPAA.den1
  Transfer Fcn1 : TransferFcn  Numerator=params.POMPAA.num2  Denominator=params.POMPAA.den2
  Transfer Fcn2 : TransferFcn  Numerator=params.POMPAA.num3  Denominator=params.POMPAA.den3
  Transport Delay : TransportDelay  DelayTime=params.POMPAA.td1
  Transport Delay1 : TransportDelay  DelayTime=params.POMPAA.td2
  Transport Delay2 : TransportDelay  DelayTime=params.POMPAA.td3
  Out1 : Outport
  wires:
  Transfer Fcn/1 -> Transport Delay/1
  Transfer Fcn1/1 -> Transport Delay1/1
  Transfer Fcn2/1 -> Transport Delay2/1
  In1/1 -> Scope2/1, Transfer Fcn/1  "omega_casA"
  In2/1 -> Scope1/1, Transfer Fcn1/1  "omega_manA"
  In3/1 -> Scope4/1, Transfer Fcn2/1  "Q"
  Sum/1 -> Scope3/1, Out1/1  "Q5A"
  Constant/1 -> Sum/4
  Transport Delay/1 -> Sum/1
  Transport Delay1/1 -> Sum/2
  Transport Delay2/1 -> Sum/3

== system System/POMPAA2 ==
  In1 : Inport
  In2 : Inport  Port=2
  In3 : Inport  Port=3
  Constant : Constant  Value=params.POMPAA.bg
  Scope{1..4} (4 alike) : Scope
  Sum : Sum  Inputs=++++
  Transfer Fcn : TransferFcn  Numerator=params.POMPAA.num1  Denominator=params.POMPAA.den1
  Transfer Fcn1 : TransferFcn  Numerator=params.POMPAA.num2  Denominator=params.POMPAA.den2
  Transfer Fcn2 : TransferFcn  Numerator=params.POMPAA.num3  Denominator=params.POMPAA.den3
  Transport Delay : TransportDelay  DelayTime=params.POMPAA.td1
  Transport Delay1 : TransportDelay  DelayTime=params.POMPAA.td2
  Transport Delay2 : TransportDelay  DelayTime=params.POMPAA.td3
  Out1 : Outport
  wires:
  Transfer Fcn/1 -> Transport Delay/1
  Transfer Fcn1/1 -> Transport Delay1/1
  Transfer Fcn2/1 -> Transport Delay2/1
  In1/1 -> Scope2/1, Transfer Fcn/1  "omega_casA"
  In2/1 -> Scope1/1, Transfer Fcn1/1  "omega_manA"
  In3/1 -> Scope4/1, Transfer Fcn2/1  "Q"
  Sum/1 -> Scope3/1, Out1/1  "Q5A"
  Constant/1 -> Sum/4
  Transport Delay/1 -> Sum/1
  Transport Delay1/1 -> Sum/2
  Transport Delay2/1 -> Sum/3

== system System/POMPAA3 ==
  In1 : Inport
  In2 : Inport  Port=2
  In3 : Inport  Port=3
  Constant : Constant  Value=params.POMPAA.bg
  Scope{1..4} (4 alike) : Scope
  Sum : Sum  Inputs=++++
  Transfer Fcn : TransferFcn  Numerator=params.POMPAA.num1  Denominator=params.POMPAA.den1
  Transfer Fcn1 : TransferFcn  Numerator=params.POMPAA.num2  Denominator=params.POMPAA.den2
  Transfer Fcn2 : TransferFcn  Numerator=params.POMPAA.num3  Denominator=params.POMPAA.den3
  Transport Delay : TransportDelay  DelayTime=params.POMPAA.td1
  Transport Delay1 : TransportDelay  DelayTime=params.POMPAA.td2
  Transport Delay2 : TransportDelay  DelayTime=params.POMPAA.td3
  Out1 : Outport
  wires:
  Transfer Fcn/1 -> Transport Delay/1
  Transfer Fcn1/1 -> Transport Delay1/1
  Transfer Fcn2/1 -> Transport Delay2/1
  In1/1 -> Scope2/1, Transfer Fcn/1  "omega_casA"
  In2/1 -> Scope1/1, Transfer Fcn1/1  "omega_manA"
  In3/1 -> Scope4/1, Transfer Fcn2/1  "Q"
  Sum/1 -> Scope3/1, Out1/1  "Q5A"
  Constant/1 -> Sum/4
  Transport Delay/1 -> Sum/1
  Transport Delay1/1 -> Sum/2
  Transport Delay2/1 -> Sum/3

== system System/POMPAA4 ==
  In1 : Inport
  In2 : Inport  Port=2
  In3 : Inport  Port=3
  Constant : Constant  Value=params.POMPAA.bg
  Scope{1..4} (4 alike) : Scope
  Sum : Sum  Inputs=++++
  Transfer Fcn : TransferFcn  Numerator=params.POMPAA.num1  Denominator=params.POMPAA.den1
  Transfer Fcn1 : TransferFcn  Numerator=params.POMPAA.num2  Denominator=params.POMPAA.den2
  Transfer Fcn2 : TransferFcn  Numerator=params.POMPAA.num3  Denominator=params.POMPAA.den3
  Transport Delay : TransportDelay  DelayTime=params.POMPAA.td1
  Transport Delay1 : TransportDelay  DelayTime=params.POMPAA.td2
  Transport Delay2 : TransportDelay  DelayTime=params.POMPAA.td3
  Out1 : Outport
  wires:
  Transfer Fcn/1 -> Transport Delay/1
  Transfer Fcn1/1 -> Transport Delay1/1
  Transfer Fcn2/1 -> Transport Delay2/1
  In1/1 -> Scope2/1, Transfer Fcn/1  "omega_casA"
  In2/1 -> Scope1/1, Transfer Fcn1/1  "omega_manA"
  In3/1 -> Scope4/1, Transfer Fcn2/1  "Q"
  Sum/1 -> Scope3/1, Out1/1  "Q5A"
  Constant/1 -> Sum/4
  Transport Delay/1 -> Sum/1
  Transport Delay1/1 -> Sum/2
  Transport Delay2/1 -> Sum/3

== system System/POMPAA5 ==
  In1 : Inport
  In2 : Inport  Port=2
  In3 : Inport  Port=3
  Constant : Constant  Value=params.POMPAA.bg
  Scope{1..4} (4 alike) : Scope
  Sum : Sum  Inputs=++++
  Transfer Fcn : TransferFcn  Numerator=params.POMPAA.num1  Denominator=params.POMPAA.den1
  Transfer Fcn1 : TransferFcn  Numerator=params.POMPAA.num2  Denominator=params.POMPAA.den2
  Transfer Fcn2 : TransferFcn  Numerator=params.POMPAA.num3  Denominator=params.POMPAA.den3
  Transport Delay : TransportDelay  DelayTime=params.POMPAA.td1
  Transport Delay1 : TransportDelay  DelayTime=params.POMPAA.td2
  Transport Delay2 : TransportDelay  DelayTime=params.POMPAA.td3
  Out1 : Outport
  wires:
  Transfer Fcn/1 -> Transport Delay/1
  Transfer Fcn1/1 -> Transport Delay1/1
  Transfer Fcn2/1 -> Transport Delay2/1
  In1/1 -> Scope2/1, Transfer Fcn/1  "omega_casA"
  In2/1 -> Scope1/1, Transfer Fcn1/1  "omega_manA"
  In3/1 -> Scope4/1, Transfer Fcn2/1  "Q"
  Sum/1 -> Scope3/1, Out1/1  "Q5A"
  Constant/1 -> Sum/4
  Transport Delay/1 -> Sum/1
  Transport Delay1/1 -> Sum/2
  Transport Delay2/1 -> Sum/3

== system System/POMPAA6 ==
  In1 : Inport
  In2 : Inport  Port=2
  In3 : Inport  Port=3
  Constant : Constant  Value=params.POMPAA.bg
  Scope{1..4} (4 alike) : Scope
  Sum : Sum  Inputs=++++
  Transfer Fcn : TransferFcn  Numerator=params.POMPAA.num1  Denominator=params.POMPAA.den1
  Transfer Fcn1 : TransferFcn  Numerator=params.POMPAA.num2  Denominator=params.POMPAA.den2
  Transfer Fcn2 : TransferFcn  Numerator=params.POMPAA.num3  Denominator=params.POMPAA.den3
  Transport Delay : TransportDelay  DelayTime=params.POMPAA.td1
  Transport Delay1 : TransportDelay  DelayTime=params.POMPAA.td2
  Transport Delay2 : TransportDelay  DelayTime=params.POMPAA.td3
  Out1 : Outport
  wires:
  Transfer Fcn/1 -> Transport Delay/1
  Transfer Fcn1/1 -> Transport Delay1/1
  Transfer Fcn2/1 -> Transport Delay2/1
  In1/1 -> Scope2/1, Transfer Fcn/1  "omega_casA"
  In2/1 -> Scope1/1, Transfer Fcn1/1  "omega_manA"
  In3/1 -> Scope4/1, Transfer Fcn2/1  "Q"
  Sum/1 -> Scope3/1, Out1/1  "Q5A"
  Constant/1 -> Sum/4
  Transport Delay/1 -> Sum/1
  Transport Delay1/1 -> Sum/2
  Transport Delay2/1 -> Sum/3

== system System/POMPAA8 ==
  In1 : Inport
  In2 : Inport  Port=2
  In3 : Inport  Port=3
  Constant : Constant  Value=params.POMPAA.bg
  Scope{1..4} (4 alike) : Scope
  Sum : Sum  Inputs=++++
  Transfer Fcn : TransferFcn  Numerator=params.POMPAA.num1  Denominator=params.POMPAA.den1
  Transfer Fcn1 : TransferFcn  Numerator=params.POMPAA.num2  Denominator=params.POMPAA.den2
  Transfer Fcn2 : TransferFcn  Numerator=params.POMPAA.num3  Denominator=params.POMPAA.den3
  Transport Delay : TransportDelay  DelayTime=params.POMPAA.td1
  Transport Delay1 : TransportDelay  DelayTime=params.POMPAA.td2
  Transport Delay2 : TransportDelay  DelayTime=params.POMPAA.td3
  Out1 : Outport
  wires:
  Transfer Fcn/1 -> Transport Delay/1
  Transfer Fcn1/1 -> Transport Delay1/1
  Transfer Fcn2/1 -> Transport Delay2/1
  In1/1 -> Scope2/1, Transfer Fcn/1  "omega_casA"
  In2/1 -> Scope1/1, Transfer Fcn1/1  "omega_manA"
  In3/1 -> Scope4/1, Transfer Fcn2/1  "Q"
  Sum/1 -> Scope3/1, Out1/1  "Q5A"
  Constant/1 -> Sum/4
  Transport Delay/1 -> Sum/1
  Transport Delay1/1 -> Sum/2
  Transport Delay2/1 -> Sum/3
